simulink model "Fuzzy_Logic_food"  (R2016a)
settings: Solver=VariableStepAuto  StartTime=0.0  StopTime=10.0  RelTol=1e-3
undefined symbols (not defined in the file or in its folder): Propina
libraries: fuzblock x1
settings Model: Creator=Daniel  LastModifiedBy=Daniel

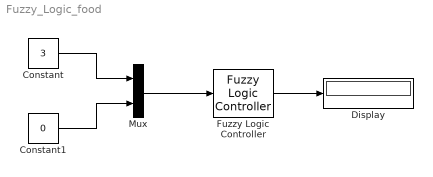
== system Fuzzy_Logic_food ==
  Constant : Constant  Value=3
  Constant1 : Constant  Value=0
  Display : Display
  Fuzzy Logic Controller : fuzblock/Fuzzy Logic  Controller  fis=[Propina]
  Mux : Mux  Inputs=2
  wires:
  Mux/1 -> Fuzzy Logic Controller/1
  Constant1/1 -> Mux/2
  Constant/1 -> Mux/1
  Fuzzy Logic Controller/1 -> Display/1
